simulink model "pvModel"  (R2022a)
settings: Solver=VariableStepAuto  StartTime=0.0  StopTime=200  RelTol=1e-3
InitFcn:
  | Isc = 9.35
  | Ki = 0.037
  | Tn = 298
  | q = 1.6e-19
  | Voc = 47.4
  | n =1.3
  | k = 1.38e-23
  | Ego = 1.1
  | Ns = 72
  | Rs = 0.39
  | Rsh = 545.82
  | NP = 3
  | NS = 4
libraries: simulink x1
settings Model: Creator=mluser  LastModifiedBy=mluser

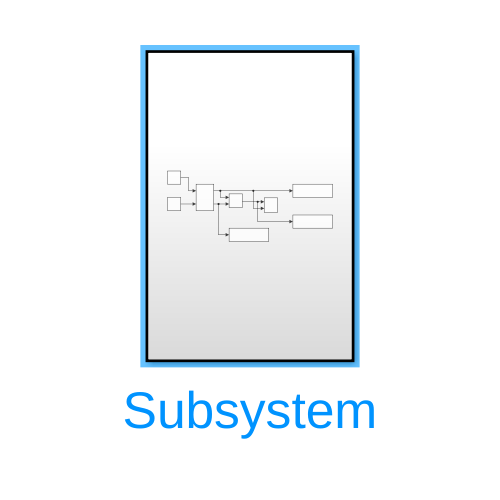
[thumbnail: Simulink's stored preview of the top-level diagram]
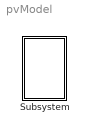
== system pvModel ==
  Subsystem : Subsystem

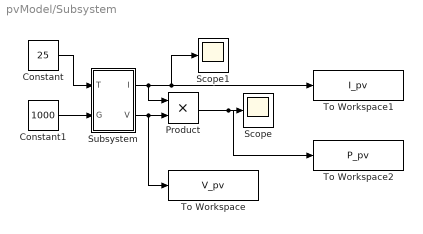
== system pvModel/Subsystem ==
  Constant : Constant  Value=25
  Constant1 : Constant  Value=1000
  Product : Product
  Scope : Scope
  Scope1 : Scope
  Subsystem : Subsystem
  To Workspace : ToWorkspace  VariableName=V_pv  SampleTime=-1
  To Workspace1 : ToWorkspace  VariableName=I_pv  SampleTime=-1
  To Workspace2 : ToWorkspace  VariableName=P_pv  SampleTime=-1
  wires:
  Constant/1 -> Subsystem/1(T)
  Constant1/1 -> Subsystem/2(G)
  Subsystem/1(I) -> Product/1, Scope1/1, To Workspace1/1
  Product/1 -> Scope/1, To Workspace2/1
  Subsystem/2(V) -> To Workspace/1, Product/2

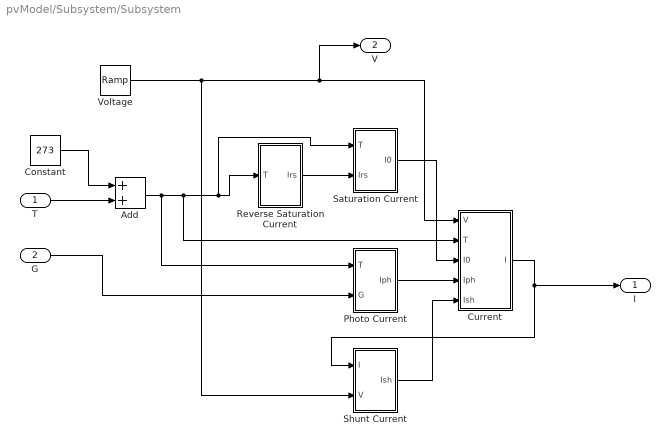
== system pvModel/Subsystem/Subsystem ==
  T : Inport
  G : Inport  Port=2
  Add : Sum
  Constant : Constant  Value=273
  Current : Subsystem
  Photo Current : Subsystem
  Reverse Saturation Current : Subsystem
  Saturation Current : Subsystem
  Shunt Current : Subsystem
  Voltage : simulink/Sources/Ramp  slope=1  start=0  InitialOutput=0
  I : Outport
  V : Outport  Port=2
  wires:
  T/1 -> Add/2
  G/1 -> Photo Current/2(G)
  Photo Current/1(Iph) -> Current/4(Iph)
  Constant/1 -> Add/1
  Shunt Current/1(Ish) -> Current/5(Ish)
  Reverse Saturation Current/1(Irs) -> Saturation Current/2(Irs)
  Add/1 -> Photo Current/1(T), Current/2(T), Saturation Current/1(T), Reverse Saturation Current/1(T)
  Saturation Current/1(I0) -> Current/3(I0)
  Current/1(I) -> I/1, Shunt Current/1(I)
  Voltage/1 -> Shunt Current/2(V), V/1, Current/1(V)

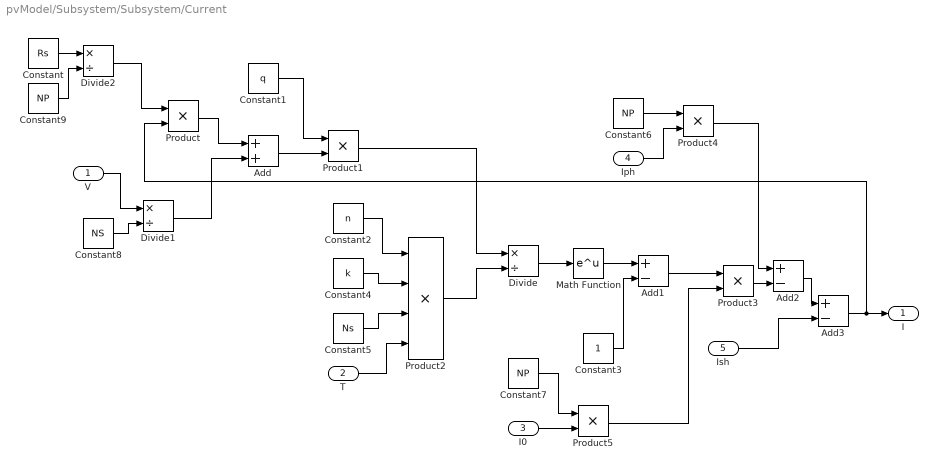
== system pvModel/Subsystem/Subsystem/Current ==
  V : Inport
  T : Inport  Port=2
  I0 : Inport  Port=3
  Iph : Inport  Port=4
  Ish : Inport  Port=5
  Add : Sum
  Add1 : Sum  Inputs=+-
  Add2 : Sum  Inputs=+-
  Add3 : Sum  Inputs=+-
  Constant : Constant  Value=Rs
  Constant1 : Constant  Value=q
  Constant2 : Constant  Value=n
  Constant3 : Constant
  Constant4 : Constant  Value=k
  Constant5 : Constant  Value=Ns
  Constant6 : Constant  Value=NP
  Constant7 : Constant  Value=NP
  Constant8 : Constant  Value=NS
  Constant9 : Constant  Value=NP
  Divide : Product  Inputs=*/
  Divide1 : Product  Inputs=*/
  Divide2 : Product  Inputs=*/
  Math Function : Math
  Product{,1,3..5} (5 alike) : Product
  Product2 : Product  Inputs=4
  I : Outport
  wires:
  Product3/1 -> Add2/2
  Add1/1 -> Product3/1
  Constant5/1 -> Product2/3
  Constant3/1 -> Add1/2
  Product1/1 -> Divide/1
  Ish/1 -> Add3/2
  Divide/1 -> Math Function/1
  Constant1/1 -> Product1/1
  Product/1 -> Add/1
  T/1 -> Product2/4
  Constant2/1 -> Product2/1
  Add/1 -> Product1/2
  Add3/1 -> I/1, Product/2
  Constant4/1 -> Product2/2
  Math Function/1 -> Add1/1
  Product2/1 -> Divide/2
  V/1 -> Divide1/1
  Add2/1 -> Add3/1
  Constant6/1 -> Product4/1
  Iph/1 -> Product4/2
  Product4/1 -> Add2/1
  Constant7/1 -> Product5/1
  I0/1 -> Product5/2
  Product5/1 -> Product3/2
  Constant8/1 -> Divide1/2
  Divide1/1 -> Add/2
  Constant/1 -> Divide2/1
  Constant9/1 -> Divide2/2
  Divide2/1 -> Product/1

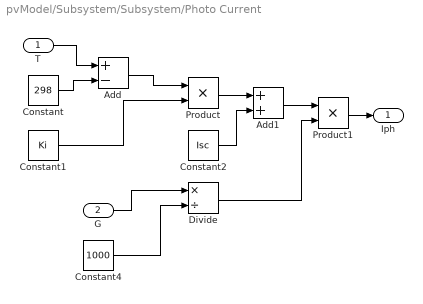
== system pvModel/Subsystem/Subsystem/Photo Current ==
  T : Inport
  G : Inport  Port=2
  Add : Sum  Inputs=+-
  Add1 : Sum
  Constant : Constant  Value=298
  Constant1 : Constant  Value=Ki
  Constant2 : Constant  Value=Isc
  Constant4 : Constant  Value=1000
  Divide : Product  Inputs=*/
  Product : Product
  Product1 : Product
  Iph : Outport
  wires:
  T/1 -> Add/1
  Constant2/1 -> Add1/2
  G/1 -> Divide/1
  Product/1 -> Add1/1
  Constant/1 -> Add/2
  Constant4/1 -> Divide/2
  Add/1 -> Product/1
  Constant1/1 -> Product/2
  Add1/1 -> Product1/1
  Divide/1 -> Product1/2
  Product1/1 -> Iph/1

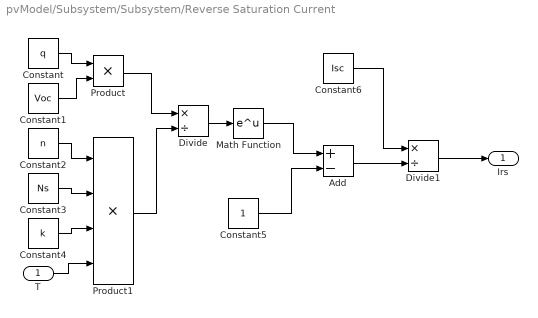
== system pvModel/Subsystem/Subsystem/Reverse Saturation Current ==
  T : Inport
  Add : Sum  Inputs=+-
  Constant : Constant  Value=q
  Constant1 : Constant  Value=Voc
  Constant2 : Constant  Value=n
  Constant3 : Constant  Value=Ns
  Constant4 : Constant  Value=k
  Constant5 : Constant
  Constant6 : Constant  Value=Isc
  Divide : Product  Inputs=*/
  Divide1 : Product  Inputs=*/
  Math Function : Math
  Product : Product
  Product1 : Product  Inputs=4
  Irs : Outport
  wires:
  Constant4/1 -> Product1/3
  Divide1/1 -> Irs/1
  Constant3/1 -> Product1/2
  Divide/1 -> Math Function/1
  Product/1 -> Divide/1
  T/1 -> Product1/4
  Add/1 -> Divide1/2
  Constant/1 -> Product/1
  Constant2/1 -> Product1/1
  Constant1/1 -> Product/2
  Constant5/1 -> Add/2
  Product1/1 -> Divide/2
  Constant6/1 -> Divide1/1
  Math Function/1 -> Add/1

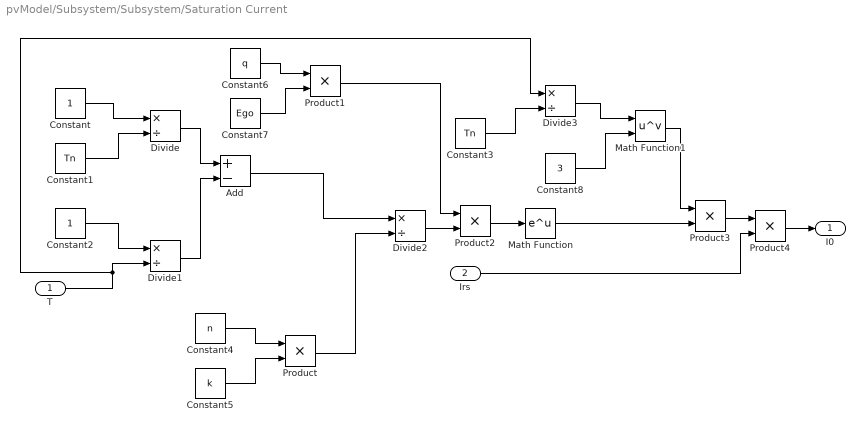
== system pvModel/Subsystem/Subsystem/Saturation Current ==
  T : Inport
  Irs : Inport  Port=2
  Add : Sum  Inputs=+-
  Constant : Constant
  Constant1 : Constant  Value=Tn
  Constant2 : Constant
  Constant3 : Constant  Value=Tn
  Constant4 : Constant  Value=n
  Constant5 : Constant  Value=k
  Constant6 : Constant  Value=q
  Constant7 : Constant  Value=Ego
  Constant8 : Constant  Value=3
  Divide{,1..3} (4 alike) : Product  Inputs=*/
  Math Function : Math
  Math Function1 : Math  Operator=pow
  Product{,1..4} (5 alike) : Product
  I0 : Outport
  wires:
  Divide/1 -> Add/1
  Constant/1 -> Divide/1
  Product2/1 -> Math Function/1
  Math Function/1 -> Product3/2
  Constant4/1 -> Product/1
  Divide3/1 -> Math Function1/1
  T/1 -> Divide1/2, Divide3/1
  Math Function1/1 -> Product3/1
  Constant8/1 -> Math Function1/2
  Constant3/1 -> Divide3/2
  Product3/1 -> Product4/1
  Constant5/1 -> Product/2
  Constant6/1 -> Product1/1
  Product1/1 -> Product2/1
  Constant1/1 -> Divide/2
  Product/1 -> Divide2/2
  Add/1 -> Divide2/1
  Constant2/1 -> Divide1/1
  Product4/1 -> I0/1
  Divide1/1 -> Add/2
  Constant7/1 -> Product1/2
  Irs/1 -> Product4/2
  Divide2/1 -> Product2/2

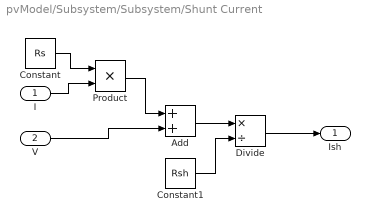
== system pvModel/Subsystem/Subsystem/Shunt Current ==
  I : Inport
  V : Inport  Port=2
  Add : Sum
  Constant : Constant  Value=Rs
  Constant1 : Constant  Value=Rsh
  Divide : Product  Inputs=*/
  Product : Product
  Ish : Outport
  wires:
  Constant1/1 -> Divide/2
  Product/1 -> Add/1
  Divide/1 -> Ish/1
  I/1 -> Product/2
  Add/1 -> Divide/1
  Constant/1 -> Product/1
  V/1 -> Add/2
